simulink model "engine_throttle_control_eric"  (R2025b)
settings: Solver=VariableStepAuto  StartTime=0.0  StopTime=10.0  RelTol=1e-3
undefined symbols (not defined in the file or in its folder): constantsSTADPOLE
settings Model: Creator=Eric  LastModifiedBy=Eric

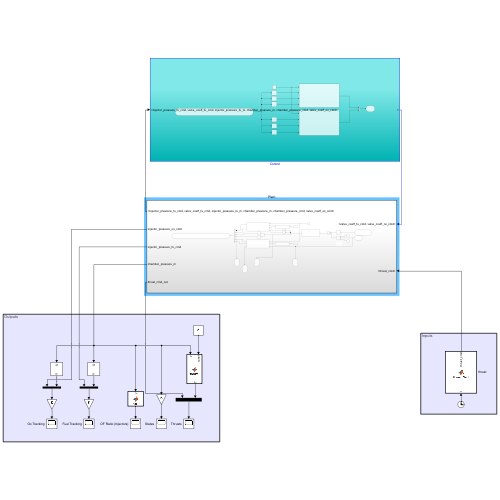
[thumbnail: Simulink's stored preview of the top-level diagram]
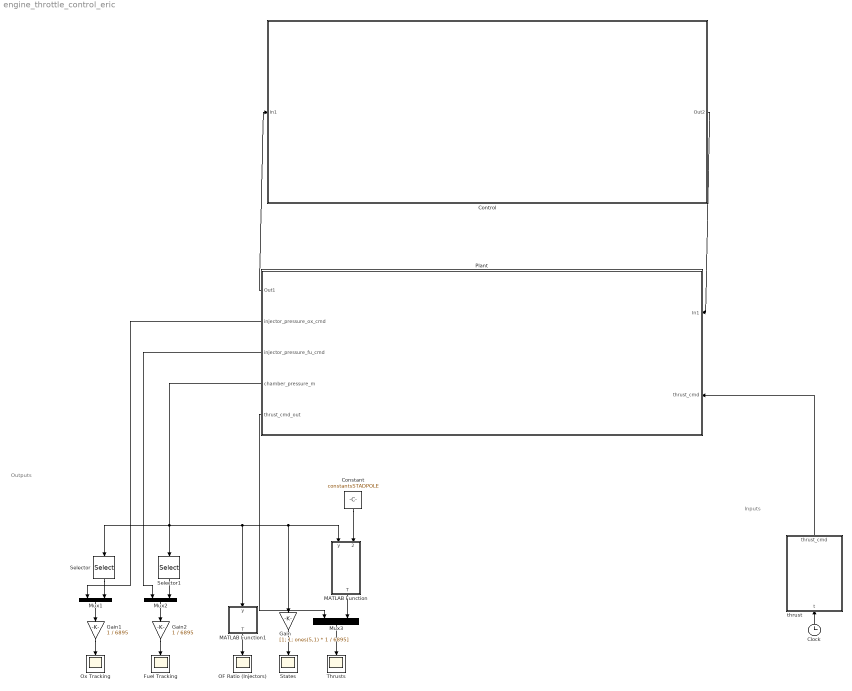
== system engine_throttle_control_eric ==
  note: Outputs
  note: Inputs
  Clock : Clock
  Constant : Constant  Value=constantsSTADPOLE  OutDataTypeStr=Bus: slBus1
  Control : Subsystem
  Fuel Tracking : Scope
      settings: ActiveDisplayYMinimum=-65.371511244894648  ActiveDisplayYMaximum=503.93015589534451  DataLoggingVariableName=ScopeData3
  Gain : Gain  Gain=[1; 1; ones(5,1) * 1 / 6895]
  Gain1 : Gain  Gain=1 / 6895
  Gain2 : Gain  Gain=1 / 6895
  MATLAB Function : MATLAB Function  TreatAsAtomicUnit=on
  MATLAB Function1 : MATLAB Function  TreatAsAtomicUnit=on
  Mux1 : Mux  Inputs=2
  Mux2 : Mux  Inputs=2
  Mux3 : Mux  Inputs=2
  OF Ratio (Injectors) : Scope
      settings: ActiveDisplayYMinimum=0  ActiveDisplayYMaximum=3  DataLoggingVariableName=ScopeData2
  Ox Tracking : Scope
      settings: ActiveDisplayYMinimum=-52.544225777854543  ActiveDisplayYMaximum=458.85039791193037  DataLoggingVariableName=ScopeData4
  Plant : Subsystem
  Selector : Selector  InputPortWidth=7  IndexOptions=Index vector (dialog)  Indices=4  OutputSizes=1
  Selector1 : Selector  InputPortWidth=7  IndexOptions=Index vector (dialog)  Indices=5  OutputSizes=1
  States : Scope
      settings: ActiveDisplayYMinimum=-5.4008603558354062E+12  ActiveDisplayYMaximum=4.8586415626429461E+13
  Thrusts : Scope
      settings: ActiveDisplayYMinimum=568.03096239670776  ActiveDisplayYMaximum=2441.1065101836757
  thrust : MATLAB Function  TreatAsAtomicUnit=on
  wires:
  thrust/1(thrust_cmd) -> Plant/2(thrust_cmd)
  Control/1(Out2) -> Plant/1(In1)
  Plant/1(Out1) -> Control/1(In1)
  Plant/2(injector_pressure_ox_cmd) -> Mux1/1
  Plant/3(injector_pressure_fu_cmd) -> Mux2/1
  Gain2/1 -> Fuel Tracking/1
  Mux1/1 -> Gain1/1
  Gain1/1 -> Ox Tracking/1
  Mux2/1 -> Gain2/1
  Selector1/1 -> Mux2/2
  Selector/1 -> Mux1/2
  MATLAB Function1/1(T) -> OF Ratio (Injectors)/1
  Plant/4(chamber_pressure_m) -> Selector/1, Gain/1, MATLAB Function/1(y), MATLAB Function1/1(y), Selector1/1
  Constant/1 -> MATLAB Function/2(const)
  MATLAB Function/1(T) -> Mux3/2
  Plant/5(thrust_cmd_out) -> Mux3/1
  Mux3/1 -> Thrusts/1
  Gain/1 -> States/1
  Clock/1 -> thrust/1(t)

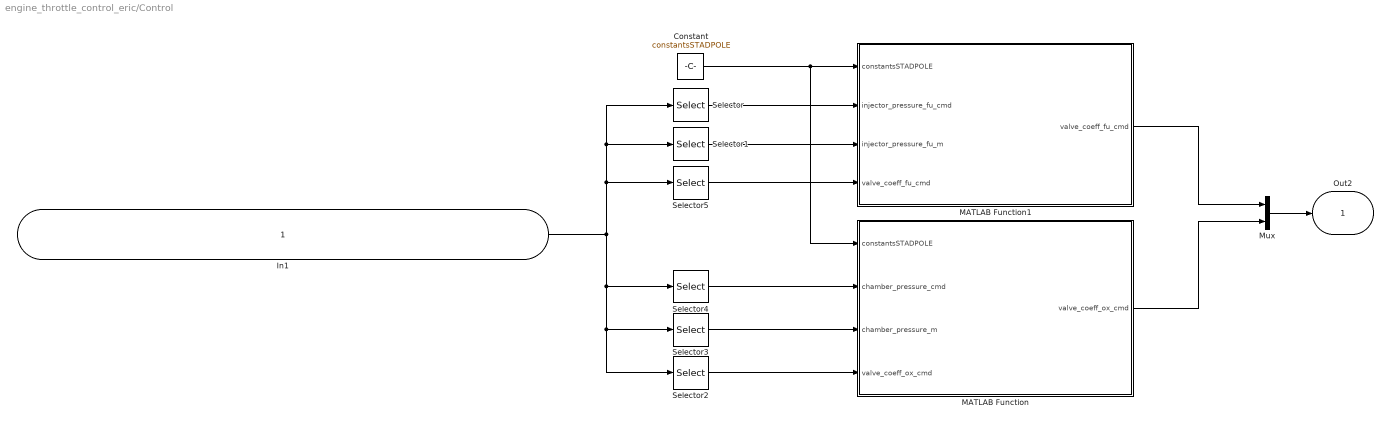
== system engine_throttle_control_eric/Control ==
  In1 : Inport
  Constant : Constant  Value=constantsSTADPOLE  OutDataTypeStr=Bus: slBus1
  MATLAB Function : MATLAB Function  TreatAsAtomicUnit=on
  MATLAB Function1 : MATLAB Function  TreatAsAtomicUnit=on
  Mux : Mux  Inputs=2
  Selector : Selector  InputPortWidth=6  IndexOptions=Index vector (dialog)  Indices=1  OutputSizes=1
  Selector1 : Selector  InputPortWidth=6  IndexOptions=Index vector (dialog)  Indices=3  OutputSizes=1
  Selector2 : Selector  InputPortWidth=6  IndexOptions=Index vector (dialog)  Indices=6  OutputSizes=1
  Selector3 : Selector  InputPortWidth=6  IndexOptions=Index vector (dialog)  Indices=4  OutputSizes=1
  Selector4 : Selector  InputPortWidth=6  IndexOptions=Index vector (dialog)  Indices=5  OutputSizes=1
  Selector5 : Selector  InputPortWidth=6  IndexOptions=Index vector (dialog)  Indices=2  OutputSizes=1
  Out2 : Outport
  wires:
  Mux/1 -> Out2/1
  Constant/1 -> MATLAB Function/1(constantsSTADPOLE), MATLAB Function1/1(constantsSTADPOLE)
  MATLAB Function/1(valve_coeff_ox_cmd) -> Mux/2
  MATLAB Function1/1(valve_coeff_fu_cmd) -> Mux/1
  Selector/1 -> MATLAB Function1/2(injector_pressure_fu_cmd)
  Selector4/1 -> MATLAB Function/2(chamber_pressure_cmd)
  Selector3/1 -> MATLAB Function/3(chamber_pressure_m)
  Selector2/1 -> MATLAB Function/4("valve_coeff_ox_cmd ")
  Selector1/1 -> MATLAB Function1/3(injector_pressure_fu_m)
  Selector5/1 -> MATLAB Function1/4("valve_coeff_fu_cmd ")
  In1/1 -> Selector5/1, Selector1/1, Selector/1, Selector2/1, Selector3/1, Selector4/1

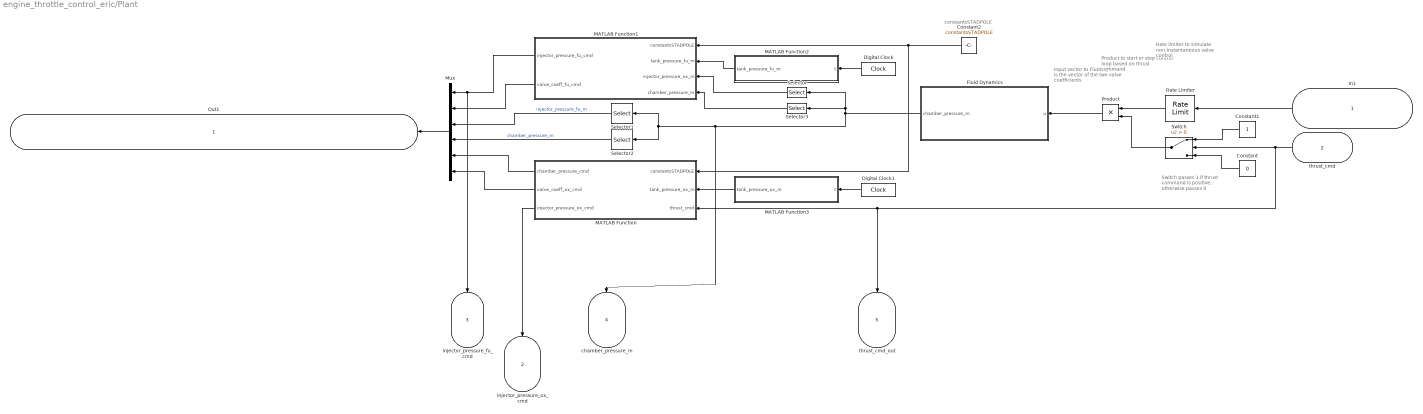
== system engine_throttle_control_eric/Plant ==
  note: constantsSTADPOLE
  note: Input vector to Fluid Dynamics is the vector of the two valve coefficients
  note: Switch passes 1 if thrust command is positive, otherwise passes 0
  note: Product to start or stop control loop based on thrust command
  note: Rate limiter to simulate non-instantaneous valve control
  In1 : Inport
  thrust_cmd : Inport  Port=2
  Constant : Constant  Value=0
  Constant1 : Constant
  Constant2 : Constant  Value=constantsSTADPOLE  OutDataTypeStr=Bus: slBus1
  Digital Clock : DigitalClock
  Digital Clock1 : DigitalClock
  Fluid Dynamics : Subsystem
  MATLAB Function : MATLAB Function  TreatAsAtomicUnit=on
  MATLAB Function1 : MATLAB Function  TreatAsAtomicUnit=on
  MATLAB Function2 : MATLAB Function  TreatAsAtomicUnit=on
  MATLAB Function3 : MATLAB Function  TreatAsAtomicUnit=on
  Mux : Mux  Inputs=6
  Product : Product
  Rate Limiter : RateLimiter  RisingSlewLimit=10^-4  FallingSlewLimit=-10^-4  SampleTimeMode=inherited
  Selector : Selector  InputPortWidth=7  IndexOptions=Index vector (dialog)  Indices=5  OutputSizes=1
  Selector1 : Selector  InputPortWidth=7  IndexOptions=Index vector (dialog)  Indices=5  OutputSizes=1
  Selector2 : Selector  InputPortWidth=7  IndexOptions=Index vector (dialog)  Indices=3  OutputSizes=1
  Selector3 : Selector  InputPortWidth=7  IndexOptions=Index vector (dialog)  Indices=3  OutputSizes=1
  Switch : Switch  Criteria=u2 > Threshold  SaturateOnIntegerOverflow=off  InputSameDT=off
  Out1 : Outport
  injector_pressure_ox_cmd : Outport  Port=2
  injector_pressure_fu_cmd : Outport  Port=3
  chamber_pressure_m : Outport  Port=4
  thrust_cmd_out : Outport  Port=5
  wires:
  Rate Limiter/1 -> Product/1
  thrust_cmd/1 -> thrust_cmd_out/1, MATLAB Function/3(thrust_cmd), Switch/2
  In1/1 -> Rate Limiter/1
  Constant/1 -> Switch/3
  Constant1/1 -> Switch/1
  Switch/1 -> Product/2
  Product/1 -> Fluid Dynamics/1(u)
  Constant2/1 -> MATLAB Function/1(constantsSTADPOLE), MATLAB Function1/1(constantsSTADPOLE)
  MATLAB Function2/1(tank_pressure_fu_m) -> MATLAB Function1/2(tank_pressure_fu_m)
  Digital Clock/1 -> MATLAB Function2/1(t)
  Digital Clock1/1 -> MATLAB Function3/1(t)
  MATLAB Function3/1(tank_pressure_ox_m) -> MATLAB Function/2(tank_pressure_ox_m)
  Selector/1 -> MATLAB Function1/3(injector_pressure_ox_m)
  Fluid Dynamics/1(chamber_pressure_m) -> Selector3/1, Selector/1, chamber_pressure_m/1, Selector2/1, Selector1/1
  MATLAB Function1/2(valve_coeff_fu_cmd) -> Mux/2
  MATLAB Function/1(chamber_pressure_cmd) -> Mux/5
  MATLAB Function/2(valve_coeff_ox_cmd) -> Mux/6
  MATLAB Function/3(injector_pressure_ox_cmd) -> injector_pressure_ox_cmd/1
  Selector1/1 -> Mux/3  "injector_pressure_fu_m"
  Mux/1 -> Out1/1
  Selector2/1 -> Mux/4  "chamber_pressure_m"
  MATLAB Function1/1(injector_pressure_fu_cmd) -> Mux/1, injector_pressure_fu_cmd/1
  Selector3/1 -> MATLAB Function1/4(chamber_pressure_m)

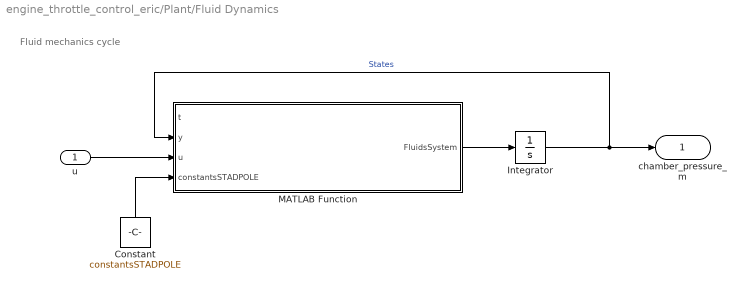
== system engine_throttle_control_eric/Plant/Fluid Dynamics ==
  note: Fluid mechanics cycle
  u : Inport
  Constant : Constant  Value=constantsSTADPOLE  OutDataTypeStr=Bus: slBus1
  Integrator : Integrator  InitialCondition=constantsSTADPOLE.init_cond
  MATLAB Function : MATLAB Function  TreatAsAtomicUnit=on
  chamber_pressure_m : Outport
  wires:
  Integrator/1 -> chamber_pressure_m/1, MATLAB Function/2(y)  "States"
  MATLAB Function/1(FluidsSystem) -> Integrator/1
  Constant/1 -> MATLAB Function/4(constantsSTADPOLE)
  u/1 -> MATLAB Function/3(u)

== matlab function engine_throttle_control_eric/Control/MATLAB Function ==
  data: constantsSTADPOLE input; valve_coeff_ox_cmd output; chamber_pressure_cmd input; chamber_pressure_m input; valve_coeff_ox_cmd input
function valve_coeff_ox_cmd  = oxygen_circuit_control (constantsSTADPOLE, chamber_pressure_cmd, chamber_pressure_m, valve_coeff_ox_cmd)

time_step = 0.001; % Add from loadtadpolesim
k_ox = 1E-11; % Add from loadtadpolesim

persistent integral_error_ox

if isempty(integral_error_ox)
        integral_error_ox = 0;
end

% No use persistent, pass error though functions

error_ox = chamber_pressure_cmd - chamber_pressure_m; % [Pa]
integral_error_ox = integral_error_ox + error_ox * time_step;
trim_ox = k_ox * integral_error_ox;
valve_coeff_ox_cmd = valve_coeff_ox_cmd + trim_ox;

== matlab function engine_throttle_control_eric/thrust ==
  data: t input; thrust_cmd output
function thrust_cmd = ThrustPlant(t)
%THRUSTPLANT 
%   random plant function for the thrust in the engine
if t < 2
    thrust_cmd = 0; %[N]
elseif mod(t,5) < 3
    thrust_cmd = 1500;
else
    thrust_cmd = 1500 - 500 * sin(mod(t,5) * pi / 2);
    
end
%cosint(t*pi/180);

end

== matlab function engine_throttle_control_eric/Control/MATLAB Function1 ==
  data: constantsSTADPOLE input; valve_coeff_fu_cmd output; injector_pressure_fu_cmd input; injector_pressure_fu_m input; valve_coeff_fu_cmd input
function valve_coeff_fu_cmd = fuel_circuit_control (constantsSTADPOLE, injector_pressure_fu_cmd, injector_pressure_fu_m, valve_coeff_fu_cmd)

time_step = 0.001; % Add from loadtadpolesim
k_fu = 1E-11; % Add from loadtadpolesim

persistent integral_error_fu

if isempty(integral_error_fu)
    integral_error_fu = 0;
end

error_fu = injector_pressure_fu_cmd - injector_pressure_fu_m; % [Pa]
integral_error_fu = integral_error_fu + error_fu * time_step;
trim_fu = k_fu * integral_error_fu;
valve_coeff_fu_cmd = valve_coeff_fu_cmd + trim_fu; % [m^3.5/kg^0.5]

== matlab function engine_throttle_control_eric/Plant/Fluid Dynamics/MATLAB Function ==
  data: t input; FluidsSystem output; y input; u input; constantsSTADPOLE input
function FluidsSystem = fluidMechanics(t, y, u, constantsSTADPOLE)
    
    % y(1)' = time rate of mass flow oxygen [kg/s^2]
    % y(2)' = time rate of mass flow fuel [kg/s^2]
    % y(3)' = time rate of chamber pressure [Pa/s]
    % y(4)' = time rate of oxygen injector press [Pa/s]
    % y(5)' = time rate of fuel injector press [Pa/s]
    % y(6)' = time rate of oxygen pressure at valve [Pa/s]
    % y(7)' = time rate of fuel pressure at valve [Pa/s]

    % y(1) = mass flow oxygen across pipe [kg/s]
    % y(2) = mass flow fuel across pipe [kg/s]
    % y(3) = chamber pressure [Pa]
    % y(4) = oxygen pressure at inj [Pa]
    % y(5) = fuel pressure at inj [Pa]
    % y(6) = oxygen pressure at valve [Pa]
    % y(7) = fuel pressure at valve [Pa]
    
    a_t= constantsSTADPOLE.a_t ; % [m^2], throat area
    
    dens_o = constantsSTADPOLE.dens_o; % [kg/m^3], liquid oxygen density, at 90 K and 1 atm
    dens_f = constantsSTADPOLE.dens_f ; % [kg/m^3], fuel density, at 293 K and 1 atm
    dens_w = constantsSTADPOLE.dens_w ; % [kg/m^3], water density
    g = constantsSTADPOLE.g ; % [m/s^2], acceleration due to gravity
    a_i_o = constantsSTADPOLE.a_i_o; % [m^2] area injector ox
    a_i_f = constantsSTADPOLE.a_i_f ; % [m^2] area injector fuel
    r = constantsSTADPOLE.r ; % [J/kg-K], specific gas constant of exhaust (molecular weight 18.8 g/mol)
    c_star = constantsSTADPOLE.c_star ; % [m/s] characteristic velocity
    of = constantsSTADPOLE.OF_target;

    c_fric = 0.03; % [unitless], line friction coefficient
    c_d_o = constantsSTADPOLE.d_coeff_ox; % [unitless], oxygen injector coefficient
    c_d_f = constantsSTADPOLE.d_coeff_fu; % [unitless], fuel injector coefficient
    l_eq_o = 7 * 0.0254; % [m], oxygen equivalent line length 
    l_eq_f = 7 * 0.0254; % [m], fuel equivalent line length 
    l_o = 120 * 0.0254; % [m], oxygen line length
    l_f = 60 * 0.0254; % [m], fuel line length
    d = (0.5 - 2 * 0.065) * 0.0254; % [m], line diameter
    v_c = 1.103170594 * 1e-3; % [m^3], chamber volume
    a_l = pi * (d / 2) ^ 2; % [m^2], line area
  
    v_l_o = a_l * l_o;
    v_l_f = a_l * l_f;
    t_o = 90; 
    t_f = 293;

    % Assume constant?
    c_v_o = 1.231e-06; %AngleToCoefficient(u(1,1));  % [m^3.5/kg^0.5], oxygen valve coefficient
    c_v_f = 1.231e-06; %AngleToCoefficient(u(2,1));  % [], fuel valve coefficient
    p_tank_o = 3.792E6; % [Pa]
    p_tank_f = 3.792E6; % [Pa]
    t_c = 3570; % [K], chamber temperature
    

    del_p_i_o = 1 / (2 * dens_o * (c_d_o * a_i_o) ^ 2); 
    del_p_l_o = 96402.2;
    del_p_i_f = 1 / (2 * dens_f * (c_d_f * a_i_f) ^ 2); 
    del_p_l_f = 2082581.1;
    

    % Momentum equations
    % massflow across pipe
    % mdot_pipe_ox = (y(4) - y(3) - del_p_l_o * y(1) * sqrt(y(1)^2 + 1e-6)) * a_l / l_o;
    % mdot_pipe_fu = (y(5) - y(3) - del_p_l_f * y(2) * sqrt(y(2)^2 + 1e-6)) * a_l / l_f;
    mddot_pipe_ox = (y(6) - y(4) - del_p_l_o * y(1) * sqrt(y(1)^2 + 1e-6)) * a_l / l_o;
    mddot_pipe_fu = (y(7) - y(5) - del_p_l_f * y(2) * sqrt(y(2)^2 + 1e-6)) * a_l / l_f;

    % Valve massflows
    ValveOX = dens_o * dens_w * (p_tank_o - y(6));
    ValveFU = dens_f * dens_w * (p_tank_f - y(7));
    mdot_valve_ox = c_v_o * ValveOX / sqrt(abs(ValveOX) + 1e2);
    mdot_valve_fu = c_v_f * ValveFU / sqrt(abs(ValveFU) + 1e2);

    % Injector massflows
    InjectorOX = 2 * dens_o *(y(4)-y(3));
    InjectorFU = 2 * dens_f * (y(5)-y(3));
    mdot_inj_ox = c_d_o * a_i_o * InjectorOX / sqrt(abs(InjectorOX)+1e2);
    mdot_inj_fu = c_d_f * a_i_f * InjectorFU / sqrt(abs(InjectorFU)+1e2);

    % Pressure at the end of the valve
    valve_ox_dot = 1e9 / (v_l_o * dens_o) * (mdot_valve_ox - y(1));
    valve_fu_dot = 1e9 / (v_l_f * dens_f) * (mdot_valve_fu - y(2));

    inj_ox_dot = 1e9 / (v_l_o*dens_o) * (y(1) - mdot_inj_ox);
    inj_fu_dot = 1e9 / (v_l_f*dens_f) * (y(2) - mdot_inj_fu);

    % Chamber Pressure equations
    pdot_chamber = (r * t_c / v_c) * (mdot_inj_ox + mdot_inj_fu - a_t * y(3) / c_star);

    % Final system
    FluidsSystem = [mddot_pipe_ox; mddot_pipe_fu; pdot_chamber; inj_ox_dot; inj_fu_dot; valve_ox_dot; valve_fu_dot];
end

== matlab function engine_throttle_control_eric/Plant/MATLAB Function ==
  data: constantsSTADPOLE input; tank_pressure_ox_m input; chamber_pressure_cmd output; valve_coeff_ox_cmd output; thrust_cmd input; injector_pressure_ox_cmd output
function [chamber_pressure_cmd, valve_coeff_ox_cmd, injector_pressure_ox_cmd] = oxygen_calculations(constantsSTADPOLE, tank_pressure_ox_m, thrust_cmd)

throat_area = constantsSTADPOLE.a_t; % [m^2]
thrust_coeff = constantsSTADPOLE.c_f; % [unitless]
char_vel = constantsSTADPOLE.c_star; % [m/s]
of_ratio = constantsSTADPOLE.OF_target; % [unitless]
rho_ox = constantsSTADPOLE.dens_o; % [kg/m^3]
discharge_coeff_ox = constantsSTADPOLE.d_coeff_ox; % [unitless],  -------------Random value just to get the code to run
orifice_area_ox = constantsSTADPOLE.a_i_o; % [m^2],  -------------Random value just to get the code to run
rho_water = constantsSTADPOLE.dens_w; % [kg/m^3]

% Valve coefficient equations
chamber_pressure_cmd = thrust_cmd / (throat_area * thrust_coeff); % [Pa]
massflow_tot_cmd = chamber_pressure_cmd * throat_area / char_vel; % [kg/s]
massflow_ox_cmd = massflow_tot_cmd * of_ratio / (of_ratio + 1); % [kg/s]
friction_pressure_drop_ox = 96402.2 * massflow_ox_cmd^2;
injector_pressure_ox_cmd = chamber_pressure_cmd + (massflow_ox_cmd ^ 2) / (2 * rho_ox * (discharge_coeff_ox * orifice_area_ox) ^ 2); % [Pa]
valve_coeff_ox_cmd = massflow_ox_cmd * sqrt(max(1 / (rho_ox * rho_water * (tank_pressure_ox_m - friction_pressure_drop_ox - injector_pressure_ox_cmd)), 0)); % [m^3.5/kg^0.5]

== matlab function engine_throttle_control_eric/Plant/MATLAB Function1 ==
  data: constantsSTADPOLE input; tank_pressure_fu_m input; injector_pressure_ox_m input; injector_pressure_fu_cmd output; valve_coeff_fu_cmd output; chamber_pressure_m input
function [injector_pressure_fu_cmd, valve_coeff_fu_cmd] = fuel_calculations(constantsSTADPOLE, tank_pressure_fu_m, injector_pressure_ox_m, chamber_pressure_m)

of_ratio = constantsSTADPOLE.OF_target; % [unitless]
rho_ox = constantsSTADPOLE.dens_o; % [kg/m^3]
rho_fu = constantsSTADPOLE.dens_f; % [kg/m^3]
discharge_coeff_ox = constantsSTADPOLE.d_coeff_ox; % [unitless],  -------------Random value just to get the code to run
discharge_coeff_fu = constantsSTADPOLE.d_coeff_fu; % [unitless],  -------------Random value just to get the code to run
orifice_area_ox = constantsSTADPOLE.a_i_o; % [m^2],  -------------Random value just to get the code to run
orifice_area_fu = constantsSTADPOLE.a_i_f; % [m^2],  -------------Random value just to get the code to run

% 150 psi at max thrust, quarter at 50%
rho_water = constantsSTADPOLE.dens_w; % [kg/m^3]

% Valve coefficient equations
delta_p_injector_ox_m = max(injector_pressure_ox_m - chamber_pressure_m, 0); % [Pa]
term_1 = sqrt(2 * delta_p_injector_ox_m * rho_ox); % [kg/m^2-s]
massflow_ox_m = discharge_coeff_ox * orifice_area_ox * term_1; % [kg/s]
massflow_fu_cmd = massflow_ox_m / of_ratio; % [kg/s]
injector_pressure_fu_cmd = chamber_pressure_m + (massflow_fu_cmd ^ 2) / (2 * rho_fu * (discharge_coeff_fu * orifice_area_fu) ^ 2); % [Pa]
friction_pressure_drop_fu = massflow_fu_cmd^2 * 2082581.1;
valve_coeff_fu_cmd = massflow_fu_cmd *  sqrt(max(1 / (rho_fu * rho_water * (tank_pressure_fu_m - friction_pressure_drop_fu - injector_pressure_fu_cmd)), 0)); % [m^3.5/kg^0.5]

== matlab function engine_throttle_control_eric/Plant/MATLAB Function2 ==
  data: t input; tank_pressure_fu_m output
function tank_pressure_fu_m = fuel_tank_pressure(t)

% Simulate fuel tank pressure, for now, assume constant at 550 psi or 3.792
% MPa

tank_pressure_fu_m = 3.792E6; % [MPa]

== matlab function engine_throttle_control_eric/Plant/MATLAB Function3 ==
  data: t input; tank_pressure_ox_m output
function tank_pressure_ox_m = oxygen_tank_pressure(t)

% Simulate oxygen tank pressure, for now, assume constant at 550 psi or 
% 3.792 MPa

tank_pressure_ox_m = 3.792E6; % [MPa]

== matlab function engine_throttle_control_eric/MATLAB Function ==
  data: y input; T output; const input
function T = thrust(y, const)

T = y(3) * const.c_f * const.a_t;

== matlab function engine_throttle_control_eric/MATLAB Function1 ==
  data: y input; T output
function T = OF(y)

T = y(1) / y(2);
